simulink model "FM_Demodulation"  (R2022b)
settings: Solver=VariableStepAuto  StartTime=0.0  StopTime=10.0  RelTol=1e-3
libraries: commsynccomp2 x2, dspfdesign x1
settings Model: Creator=Sahaj Singh  LastModifiedBy=Sahaj Singh

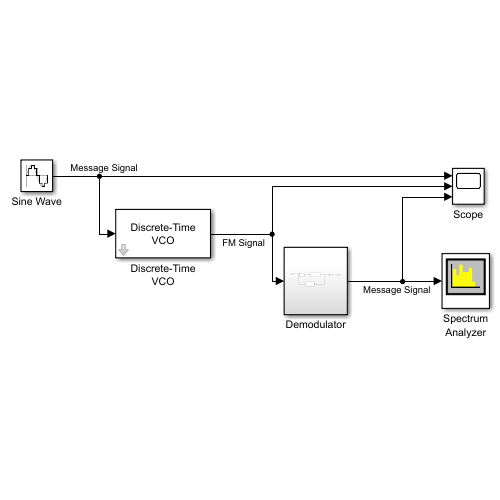
[thumbnail: Simulink's stored preview of the top-level diagram]
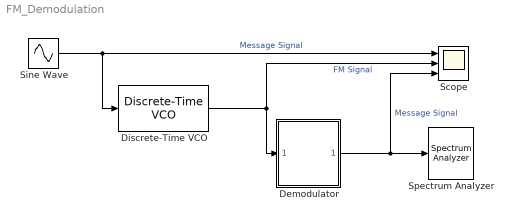
== system FM_Demodulation ==
  Demodulator : Subsystem
  Discrete-Time VCO : commsynccomp2/Discrete-Time VCO  Ac=1  Fc=10000  Kc=2500  Ph=0  ts=0.00001
  Scope : Scope  NumInputPorts=3
  Sine Wave : Sin  Frequency=12566.370614  SampleTime=0.00001
  Spectrum Analyzer : SpectrumAnalyzer
  wires:
  Sine Wave/1 -> Scope/1, Discrete-Time VCO/1  "Message Signal"
  Discrete-Time VCO/1 -> Demodulator/1(FM Signal Input), Scope/2  "FM Signal"
  Demodulator/1(Amplified Message Signal Output) -> Scope/3, Spectrum Analyzer/1  "Message Signal"

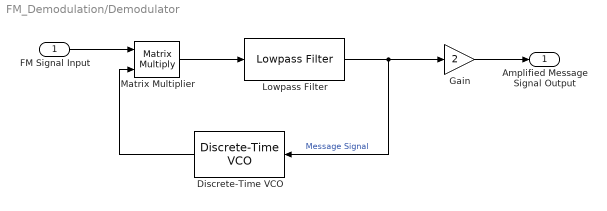
== system FM_Demodulation/Demodulator ==
  FM Signal Input : Inport
  Discrete-Time VCO : commsynccomp2/Discrete-Time VCO  Ac=1  Fc=10000  Kc=2500  Ph=0  ts=0.00001
  Gain : Gain  Gain=2
  Lowpass Filter : dspfdesign/Lowpass Filter  FilterType=FIR  DesignForMinimumOrder=on  FilterOrder=50  PassbandFrequency=2500  StopbandFrequency=3000  PassbandRipple=0.1  StopbandAttenuation=80  InheritSampleRate=off  SampleRate=100000  SimulateUsing=Interpreted execution  roundingMode=Floor  coeffsDataTypeStr=fixdt(1,16)
  Matrix Multiplier : Product  Multiplication=Matrix(*)
  Amplified Message Signal Output : Outport
  wires:
  FM Signal Input/1 -> Matrix Multiplier/1
  Matrix Multiplier/1 -> Lowpass Filter/1
  Lowpass Filter/1 -> Discrete-Time VCO/1, Gain/1  "Message Signal"
  Discrete-Time VCO/1 -> Matrix Multiplier/2
  Gain/1 -> Amplified Message Signal Output/1
